simulink model "main_sim"  (R2025b)
settings: Solver=FixedStepAuto  StartTime=0.0  StopTime=100  FixedStep=sample_time  RelTol=1e-3
values from neighbouring files (symbols this model uses):
  A_cut_in = 0.03    [matlab.mat]    (also in params.m = 0.16)
  att_ctrl_time = 0.004    [matlab.mat]    (also in params.m)
  control_allocator_matrix = [0 0 0.106752068321 1.89324793168 0 1 0 0 1 0 0 0 ... (16 elements, 4x4)]    [matlab.mat]    (also in params.m = inv(control_effectiveness_matrix))
  f_xy_tf = load("f_xy_tf.mat").tf1    [params.m]
  initial_euler = [0 0.1 0]    [matlab.mat]    (also in params.m = [0, 0, 0])
  K_coeff = 0.84020150191    [matlab.mat]    (also in params.m = 0.348193185773)
  mav_mass = 0.6    [matlab.mat]    (also in params.m)
  phase_lag = 0    [matlab.mat]    (also in params.m)
  rate_ctrl_time = 0.001    [matlab.mat]    (also in params.m)
  thrust_coeff_bot = 10    [matlab.mat]    (also in params.m = 10.9837)
  thrust_coeff_top = 8.4216    [matlab.mat]    (also in params.m = 9.346)
  top_motor_arm = [0 0 0.1]    [matlab.mat]    (also in params.m = [0, 0, 0.1])
  torque_coeff_bot = 0.1    [matlab.mat]    (also in params.m = 0.1455)
  torque_coeff_top = 1.7735    [matlab.mat]    (also in params.m = 0.2051)
undefined symbols (not defined in the file or in its folder): fractalcoef, SampleTime
libraries: aerolibutil x3, sharedtransform x2, simulink_extras x1, aerolibobsolete x1, matrix_library x1, uavutilslib x1, sensorgpslib x1, mspsensorlib x1
settings Model: Creator=tommy  LastModifiedBy=tommy
settings OptimizationCC: DefaultParameterBehavior=Inlined  UseDivisionForNetSlopeComputation=on  GainParamInheritBuiltInType=on  UseFloatMulNetSlope=on  InlineInvariantSignals=on  EnhancedBackFolding=on  BooleansAsBitfields=on  PassReuseOutputArgsAs=Individual arguments  StateBitsets=on  DataBitsets=on  ZeroExternalMemoryAtStartup=off  ZeroInternalMemoryAtStartup=off  NoFixptDivByZeroProtection=on  EfficientFloat2IntCast=on  LifeSpan=1  OptimizeBlockOrder=speed  DifferentSizesBufferReuse=on  EfficientTunableParamExpr=on
settings DebuggingCC: ParameterTunabilityLossMsg=error
settings HardwareCC: ProdBitPerPointer=32.0  ProdBitPerSizeT=32.0  ProdBitPerPtrDiffT=32.0  ProdLargestAtomicInteger=Long  ProdLargestAtomicFloat=Double  ProdWordSize=32.0  ProdLongLongMode=on  ProdHWDeviceType=ARM Compatible->ARM Cortex-M
settings SFSimCC: MATLABDynamicMemAlloc=off  SimTargetLang=C++  SimDLTargetLibrary=mkl-dnn
settings RTWCC: SystemTargetFile=ert.tlc  TemplateMakefile=ert_default_tmf  TargetLang=C++  Description=Embedded Coder
settings CodeAppCC: ForceParamTrailComments=on  IgnoreCustomStorageClasses=off  OperatorAnnotations=on  SimulinkDataObjDesc=on  SFDataObjDesc=on  CustomSymbolStrGlobalVar=rt$N$M  CustomSymbolStrType=$N$M  CustomSymbolStrFcn=$N$M$F  CustomSymbolStrMacro=$N$M  InsertBlockDesc=on
settings ERTTargetCC: RootIOFormat=Structure reference  ERTCustomFileTemplate=example_file_process.tlc  ERTFilePackagingFormat=CompactWithDataFile  TargetLangStandard=C++11 (ISO)  GenerateSampleERTMain=on  IncludeMdlTerminateFcn=off  CombineSignalStateStructs=on  SuppressErrorStatus=on  SupportAbsoluteTime=off  CodeInterfacePackaging=C++ class  SupportComplex=off

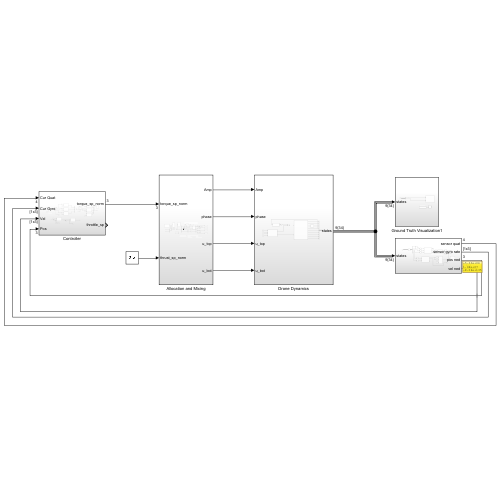
[thumbnail: Simulink's stored preview of the top-level diagram]
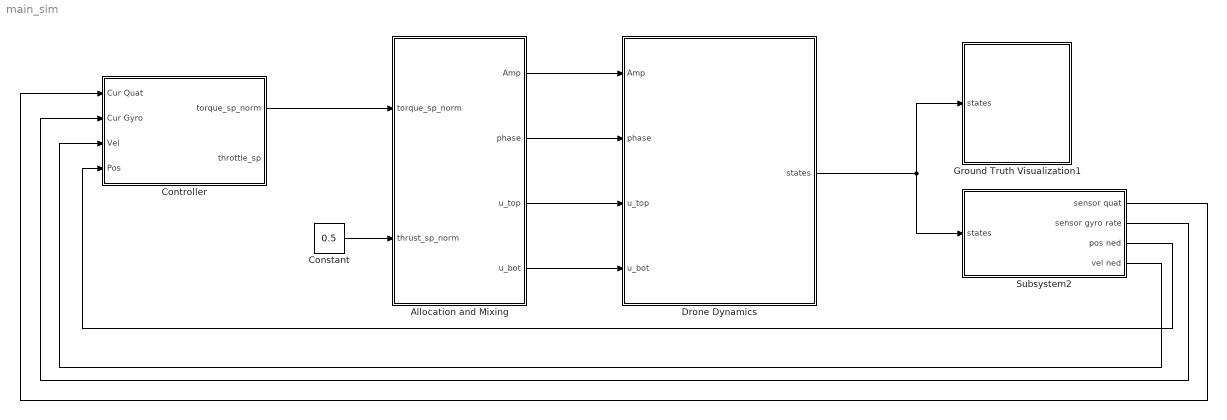
== system main_sim ==
  Allocation and Mixing : Subsystem
  Constant : Constant  Value=0.5
  Controller : Subsystem
  Drone Dynamics : Subsystem
  Ground Truth Visualization1 : Subsystem
  Subsystem2 : Subsystem
  wires:
  Controller/1(torque_sp_norm) -> Allocation and Mixing/1(torque_sp_norm)
  Drone Dynamics/1(states) -> Ground Truth Visualization1/1(states), Subsystem2/1(states)
  Allocation and Mixing/2(phase) -> Drone Dynamics/2(phase)
  Allocation and Mixing/3(u_top) -> Drone Dynamics/3(u_top)
  Allocation and Mixing/4(u_bot) -> Drone Dynamics/4(u_bot)
  Subsystem2/2(sensor gyro rate) -> Controller/2(Cur Gyro)
  Subsystem2/1(sensor quat) -> Controller/1(Cur Quat)
  Allocation and Mixing/1(Amp) -> Drone Dynamics/1(Amp)
  Subsystem2/4(vel ned) -> Controller/3(Vel)
  Subsystem2/3(pos ned) -> Controller/4(Pos)
  Constant/1 -> Allocation and Mixing/2(thrust_sp_norm)

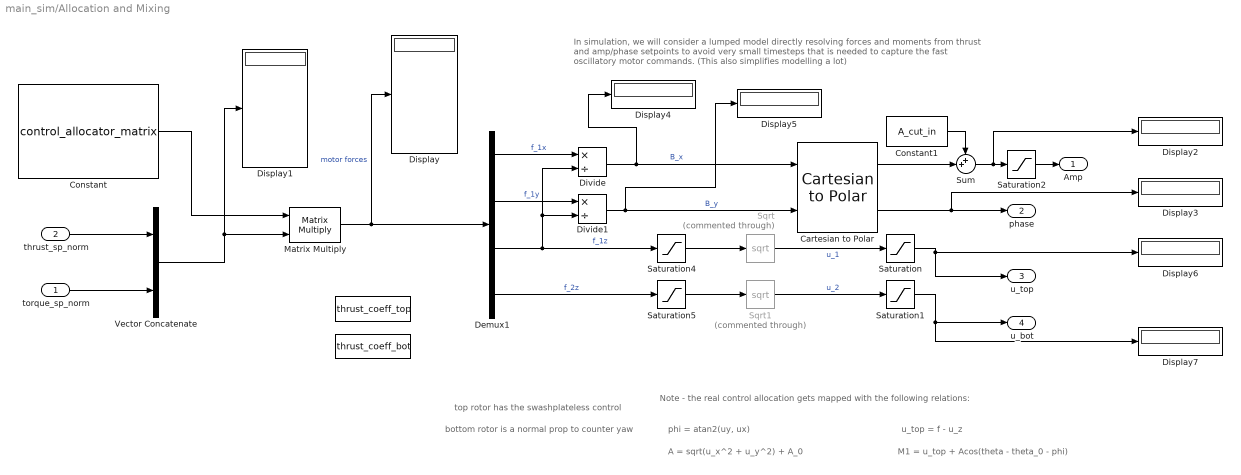
== system main_sim/Allocation and Mixing ==
  note: u_top = f - u_z
  note: In simulation, we will consider a lumped model directly resolving forces and moments from thrust and amp/phase setpoints to avoid very small timesteps that is needed to capture the fast oscillatory motor commands. (This also simplifies modelling a lot)
  note: phi = atan2(uy, ux)
  note: A = sqrt(u_x^2 + u_y^2) + A_0
  note: top rotor has the swashplateless control
  note: bottom rotor is a normal prop to counter yaw
  note: Note - the real control allocation gets mapped with the following relations:
  note: M1 = u_top + Acos(theta - theta_0 - phi)
  torque_sp_norm : Inport
  thrust_sp_norm : Inport  Port=2
  " " : Constant  Value=thrust_coeff_top
  "  " : Constant  Value=thrust_coeff_bot
  Cartesian to Polar : simulink_extras/Transformations/Cartesian to Polar
  Constant : Constant  Value=control_allocator_matrix
  Constant1 : Constant  Value=A_cut_in
  Demux1 : Demux
  Display{,1..7} (8 alike) : Display
  Divide : Product  Inputs=*/
  Divide1 : Product  Inputs=*/
  Matrix Multiply : Product  Multiplication=Matrix(*)
  Saturation : Saturate  UpperLimit=1  LowerLimit=0
  Saturation1 : Saturate  UpperLimit=1  LowerLimit=0
  Saturation2 : Saturate  UpperLimit=0.3
  Saturation4 : Saturate  UpperLimit=inf  LowerLimit=0
  Saturation5 : Saturate  UpperLimit=inf  LowerLimit=0
  Sqrt : Sqrt  Commented=through
  Sqrt1 : Sqrt  Commented=through
  Sum : Sum  Inputs=++|
  Vector Concatenate : Concatenate
  Amp : Outport
  phase : Outport  Port=2
  u_top : Outport  Port=3
  u_bot : Outport  Port=4
  wires:
  Divide/1 -> Display4/1, Cartesian to Polar/1  "B_x"
  Divide1/1 -> Display5/1, Cartesian to Polar/2  "B_y"
  Cartesian to Polar/2 -> Display3/1, phase/1
  Saturation/1 -> u_top/1, Display6/1
  Saturation1/1 -> Display7/1, u_bot/1
  Demux1/1 -> Divide/1  "f_1x"
  Demux1/2 -> Divide1/1  "f_1y"
  Demux1/3 -> Divide/2, Divide1/2, Saturation4/1  "f_1z"
  Demux1/4 -> Saturation5/1  "f_2z"
  Sqrt/1 -> Saturation/1  "u_1"
  Sqrt1/1 -> Saturation1/1  "u_2"
  torque_sp_norm/1 -> Vector Concatenate/2
  Constant/1 -> Matrix Multiply/1
  thrust_sp_norm/1 -> Vector Concatenate/1
  Vector Concatenate/1 -> Display1/1, Matrix Multiply/2
  Matrix Multiply/1 -> Display/1, Demux1/1  "motor forces"
  Sum/1 -> Saturation2/1, Display2/1
  Cartesian to Polar/1 -> Sum/2
  Constant1/1 -> Sum/1
  Saturation4/1 -> Sqrt/1
  Saturation5/1 -> Sqrt1/1
  Saturation2/1 -> Amp/1

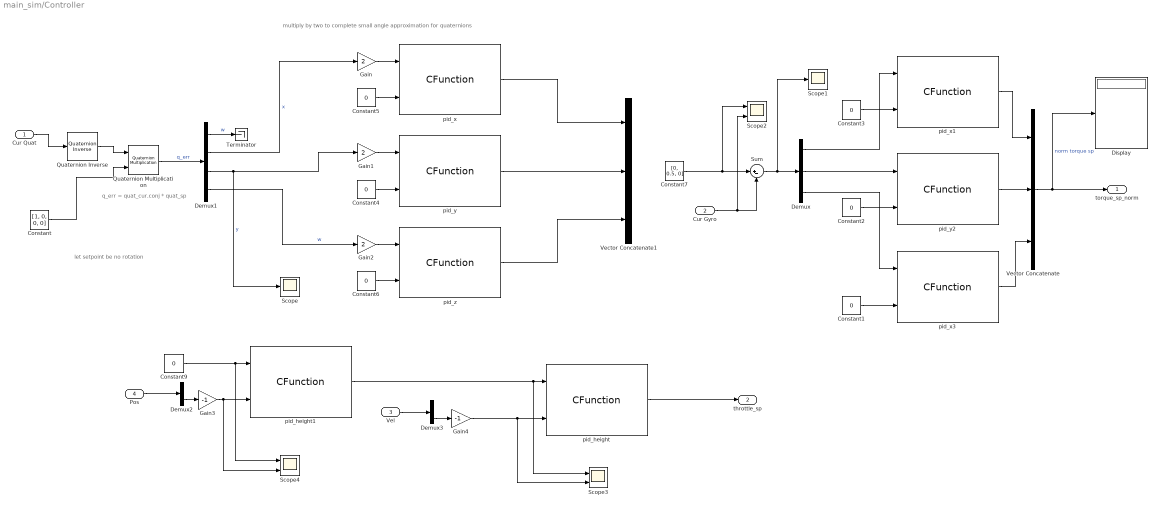
== system main_sim/Controller ==
  note: let setpoint be no rotation
  note: q_err = quat_cur.conj * quat_sp
  note: multiply by two to complete small angle approximation for quaternions
  Cur Quat : Inport
  Cur Gyro : Inport  Port=2
  Vel : Inport  Port=3
  Pos : Inport  Port=4
  Constant : Constant  Value=[1, 0, 0, 0]
  Constant{1..6,9} (7 alike) : Constant  Value=0
  Constant7 : Constant  Value=[0, 0.5, 0]
  Demux : Demux  Outputs=3
  Demux1 : Demux
  Demux2 : Demux  Outputs=3
  Demux3 : Demux  Outputs=3
  Display : Display
  Gain : Gain  Gain=2
  Gain1 : Gain  Gain=2
  Gain2 : Gain  Gain=2
  Gain3 : Gain  Gain=-1
  Gain4 : Gain  Gain=-1
  Quaternion Inverse : aerolibutil/Quaternion Inverse
  Quaternion Multiplication : aerolibutil/Quaternion Multiplication
  Scope : Scope
      settings: ActiveDisplayYMinimum=-0.059979169270678333  ActiveDisplayYMaximum=-0.039979169270678329  DataLoggingVariableName=ScopeData2
  Scope1 : Scope
      settings: ActiveDisplayYMinimum=-0.0842010868455836  ActiveDisplayYMaximum=-0.046176733596834114  DataLoggingVariableName=ScopeData3
  Scope2 : Scope  NumInputPorts=2
      settings: ActiveDisplayYMinimum=-2.2288514415526066  ActiveDisplayYMaximum=0.61387387896787893  DataLoggingVariableName=ScopeData4
  Scope3 : Scope  NumInputPorts=2
      settings: ActiveDisplayYMinimum=-1.8084870099704817  ActiveDisplayYMaximum=0.34454279174231495  DataLoggingVariableName=ScopeData6
  Scope4 : Scope  NumInputPorts=2
      settings: ActiveDisplayYMinimum=-2.2966254517668858  ActiveDisplayYMaximum=2.4973444218048826  DataLoggingVariableName=ScopeData7
  Sum : Sum  Inputs=|+-
  Terminator : Terminator
  Vector Concatenate : Concatenate  NumInputs=3
  Vector Concatenate1 : Concatenate  NumInputs=3
  pid_height : CFunction  OutputCode=|  StartCode=obj_ptr = create_pid((float)Ts, (float)max, (float)min, (float)K, (float)Kp, (float)Ki, (float)Kd, (float)clamp, (float)alpha);  TerminateCode=|  CodegenOutputCode=|  CodegenStartCode=obj_ptr = create_pid((float)Ts, (float)max, (float)min, (float)K, (float)Kp, (float)Ki, (float)Kd, (float)clamp, (float)alpha);  CodegenTerminateCode=|  SampleTime=SampleTime  SimCustomHeaderFile="#include \"cpp/pid_wrap.hpp\""  SimCustomSourceFile=pid_wrap.cpp  CustomHeaderFile="#include \"cpp/pid_wrap.hpp\""  CustomSourceFile=pid_wrap.cpp  CustomCodeIsMultiInstantiable=on  Ts=att_ctrl_time  max=1  min=0.1  K=1  Kp=0.3  Ki=0.6  Kd=0  clamp=0.8  alpha=0  SampleTime=att_ctrl_time
      OutputCode=|
      | if (obj_ptr != 0) {
      |     out = (double)run_pid(obj_ptr, (float)setpoint, (float)measurement);
      | }
      TerminateCode=|
      | if (obj_ptr != 0) {
      |     delete_pid(obj_ptr);
      |     obj_ptr = 0;
      | }
      CodegenOutputCode=|
      | if (obj_ptr != 0) {
      |     out = (double)run_pid(obj_ptr, (float)setpoint, (float)measurement);
      | }
      CodegenTerminateCode=|
      | if (obj_ptr != 0) {
      |     delete_pid(obj_ptr);
      |     obj_ptr = 0;
      | }
  pid_height1 : CFunction  OutputCode=|  StartCode=obj_ptr = create_pid((float)Ts, (float)max, (float)min, (float)K, (float)Kp, (float)Ki, (float)Kd, (float)clamp, (float)alpha);  TerminateCode=|  CodegenOutputCode=|  CodegenStartCode=obj_ptr = create_pid((float)Ts, (float)max, (float)min, (float)K, (float)Kp, (float)Ki, (float)Kd, (float)clamp, (float)alpha);  CodegenTerminateCode=|  SampleTime=SampleTime  SimCustomHeaderFile="#include \"cpp/pid_wrap.hpp\""  SimCustomSourceFile=pid_wrap.cpp  CustomHeaderFile="#include \"cpp/pid_wrap.hpp\""  CustomSourceFile=pid_wrap.cpp  CustomCodeIsMultiInstantiable=on  Ts=att_ctrl_time  max=5  min=-5  K=1  Kp=0.2  Ki=0  Kd=0  clamp=0.8  alpha=0  SampleTime=att_ctrl_time
      OutputCode=|
      | if (obj_ptr != 0) {
      |     out = (double)run_pid(obj_ptr, (float)setpoint, (float)measurement);
      | }
      TerminateCode=|
      | if (obj_ptr != 0) {
      |     delete_pid(obj_ptr);
      |     obj_ptr = 0;
      | }
      CodegenOutputCode=|
      | if (obj_ptr != 0) {
      |     out = (double)run_pid(obj_ptr, (float)setpoint, (float)measurement);
      | }
      CodegenTerminateCode=|
      | if (obj_ptr != 0) {
      |     delete_pid(obj_ptr);
      |     obj_ptr = 0;
      | }
  pid_x : CFunction  OutputCode=|  StartCode=obj_ptr = create_pid((float)Ts, (float)max, (float)min, (float)K, (float)Kp, (float)Ki, (float)Kd, (float)clamp, (float)alpha);  TerminateCode=|  CodegenOutputCode=|  CodegenStartCode=obj_ptr = create_pid((float)Ts, (float)max, (float)min, (float)K, (float)Kp, (float)Ki, (float)Kd, (float)clamp, (float)alpha);  CodegenTerminateCode=|  SampleTime=SampleTime  SimCustomHeaderFile="#include \"cpp/pid_wrap.hpp\""  SimCustomSourceFile=pid_wrap.cpp  CustomHeaderFile="#include \"cpp/pid_wrap.hpp\""  CustomSourceFile=pid_wrap.cpp  CustomCodeIsMultiInstantiable=on  Ts=att_ctrl_time  max=1  min=-1  K=1  Kp=0.1  Ki=0  Kd=0  clamp=0  alpha=0  SampleTime=att_ctrl_time
      OutputCode=|
      | if (obj_ptr != 0) {
      |     out = (double)run_pid(obj_ptr, (float)setpoint, (float)measurement);
      | }
      TerminateCode=|
      | if (obj_ptr != 0) {
      |     delete_pid(obj_ptr);
      |     obj_ptr = 0;
      | }
      CodegenOutputCode=|
      | if (obj_ptr != 0) {
      |     out = (double)run_pid(obj_ptr, (float)setpoint, (float)measurement);
      | }
      CodegenTerminateCode=|
      | if (obj_ptr != 0) {
      |     delete_pid(obj_ptr);
      |     obj_ptr = 0;
      | }
  pid_x1 : CFunction  OutputCode=|  StartCode=obj_ptr = create_pid((float)Ts, (float)max, (float)min, (float)K, (float)Kp, (float)Ki, (float)Kd, (float)clamp, (float)alpha);  TerminateCode=|  CodegenOutputCode=|  CodegenStartCode=obj_ptr = create_pid((float)Ts, (float)max, (float)min, (float)K, (float)Kp, (float)Ki, (float)Kd, (float)clamp, (float)alpha);  CodegenTerminateCode=|  SampleTime=SampleTime  SimCustomHeaderFile="#include \"cpp/pid_wrap.hpp\""  SimCustomSourceFile=pid_wrap.cpp  CustomHeaderFile="#include \"cpp/pid_wrap.hpp\""  CustomSourceFile=pid_wrap.cpp  CustomCodeIsMultiInstantiable=on  Ts=rate_ctrl_time  max=1  min=-1  K=1  Kp=0.02  Ki=0  Kd=0  clamp=0  alpha=0  SampleTime=rate_ctrl_time
      OutputCode=|
      | if (obj_ptr != 0) {
      |     out = (double)run_pid(obj_ptr, (float)setpoint, (float)measurement);
      | }
      TerminateCode=|
      | if (obj_ptr != 0) {
      |     delete_pid(obj_ptr);
      |     obj_ptr = 0;
      | }
      CodegenOutputCode=|
      | if (obj_ptr != 0) {
      |     out = (double)run_pid(obj_ptr, (float)setpoint, (float)measurement);
      | }
      CodegenTerminateCode=|
      | if (obj_ptr != 0) {
      |     delete_pid(obj_ptr);
      |     obj_ptr = 0;
      | }
  pid_x3 : CFunction  OutputCode=|  StartCode=obj_ptr = create_pid((float)Ts, (float)max, (float)min, (float)K, (float)Kp, (float)Ki, (float)Kd, (float)clamp, (float)alpha);  TerminateCode=|  CodegenOutputCode=|  CodegenStartCode=obj_ptr = create_pid((float)Ts, (float)max, (float)min, (float)K, (float)Kp, (float)Ki, (float)Kd, (float)clamp, (float)alpha);  CodegenTerminateCode=|  SampleTime=SampleTime  SimCustomHeaderFile="#include \"cpp/pid_wrap.hpp\""  SimCustomSourceFile=pid_wrap.cpp  CustomHeaderFile="#include \"cpp/pid_wrap.hpp\""  CustomSourceFile=pid_wrap.cpp  CustomCodeIsMultiInstantiable=on  Ts=rate_ctrl_time  max=1  min=-1  K=1  Kp=0.1  Ki=0.3  Kd=0  clamp=0.3  alpha=0  SampleTime=rate_ctrl_time
      OutputCode=|
      | if (obj_ptr != 0) {
      |     out = (double)run_pid(obj_ptr, (float)setpoint, (float)measurement);
      | }
      TerminateCode=|
      | if (obj_ptr != 0) {
      |     delete_pid(obj_ptr);
      |     obj_ptr = 0;
      | }
      CodegenOutputCode=|
      | if (obj_ptr != 0) {
      |     out = (double)run_pid(obj_ptr, (float)setpoint, (float)measurement);
      | }
      CodegenTerminateCode=|
      | if (obj_ptr != 0) {
      |     delete_pid(obj_ptr);
      |     obj_ptr = 0;
      | }
  pid_y : CFunction  OutputCode=|  StartCode=obj_ptr = create_pid((float)Ts, (float)max, (float)min, (float)K, (float)Kp, (float)Ki, (float)Kd, (float)clamp, (float)alpha);  TerminateCode=|  CodegenOutputCode=|  CodegenStartCode=obj_ptr = create_pid((float)Ts, (float)max, (float)min, (float)K, (float)Kp, (float)Ki, (float)Kd, (float)clamp, (float)alpha);  CodegenTerminateCode=|  SampleTime=SampleTime  SimCustomHeaderFile="#include \"cpp/pid_wrap.hpp\""  SimCustomSourceFile=pid_wrap.cpp  CustomHeaderFile="#include \"cpp/pid_wrap.hpp\""  CustomSourceFile=pid_wrap.cpp  CustomCodeIsMultiInstantiable=on  Ts=att_ctrl_time  max=1  min=-1  K=1  Kp=0.5  Ki=0  Kd=0  clamp=0  alpha=0  SampleTime=att_ctrl_time
      OutputCode=|
      | if (obj_ptr != 0) {
      |     out = (double)run_pid(obj_ptr, (float)setpoint, (float)measurement);
      | }
      TerminateCode=|
      | if (obj_ptr != 0) {
      |     delete_pid(obj_ptr);
      |     obj_ptr = 0;
      | }
      CodegenOutputCode=|
      | if (obj_ptr != 0) {
      |     out = (double)run_pid(obj_ptr, (float)setpoint, (float)measurement);
      | }
      CodegenTerminateCode=|
      | if (obj_ptr != 0) {
      |     delete_pid(obj_ptr);
      |     obj_ptr = 0;
      | }
  pid_y2 : CFunction  OutputCode=|  StartCode=obj_ptr = create_pid((float)Ts, (float)max, (float)min, (float)K, (float)Kp, (float)Ki, (float)Kd, (float)clamp, (float)alpha);  TerminateCode=|  CodegenOutputCode=|  CodegenStartCode=obj_ptr = create_pid((float)Ts, (float)max, (float)min, (float)K, (float)Kp, (float)Ki, (float)Kd, (float)clamp, (float)alpha);  CodegenTerminateCode=|  SampleTime=SampleTime  SimCustomHeaderFile="#include \"cpp/pid_wrap.hpp\""  SimCustomSourceFile=pid_wrap.cpp  CustomHeaderFile="#include \"cpp/pid_wrap.hpp\""  CustomSourceFile=pid_wrap.cpp  CustomCodeIsMultiInstantiable=on  Ts=rate_ctrl_time  max=1  min=-1  K=1  Kp=0.02  Ki=0  Kd=0  clamp=0  alpha=0  SampleTime=rate_ctrl_time
      OutputCode=|
      | if (obj_ptr != 0) {
      |     out = (double)run_pid(obj_ptr, (float)setpoint, (float)measurement);
      | }
      TerminateCode=|
      | if (obj_ptr != 0) {
      |     delete_pid(obj_ptr);
      |     obj_ptr = 0;
      | }
      CodegenOutputCode=|
      | if (obj_ptr != 0) {
      |     out = (double)run_pid(obj_ptr, (float)setpoint, (float)measurement);
      | }
      CodegenTerminateCode=|
      | if (obj_ptr != 0) {
      |     delete_pid(obj_ptr);
      |     obj_ptr = 0;
      | }
  pid_z : CFunction  OutputCode=|  StartCode=obj_ptr = create_pid((float)Ts, (float)max, (float)min, (float)K, (float)Kp, (float)Ki, (float)Kd, (float)clamp, (float)alpha);  TerminateCode=|  CodegenOutputCode=|  CodegenStartCode=obj_ptr = create_pid((float)Ts, (float)max, (float)min, (float)K, (float)Kp, (float)Ki, (float)Kd, (float)clamp, (float)alpha);  CodegenTerminateCode=|  SampleTime=SampleTime  SimCustomHeaderFile="#include \"cpp/pid_wrap.hpp\""  SimCustomSourceFile=pid_wrap.cpp  CustomHeaderFile="#include \"cpp/pid_wrap.hpp\""  CustomSourceFile=pid_wrap.cpp  CustomCodeIsMultiInstantiable=on  Ts=att_ctrl_time  max=1  min=-1  K=1  Kp=0.1  Ki=0  Kd=0  clamp=0  alpha=0  SampleTime=att_ctrl_time
      OutputCode=|
      | if (obj_ptr != 0) {
      |     out = (double)run_pid(obj_ptr, (float)setpoint, (float)measurement);
      | }
      TerminateCode=|
      | if (obj_ptr != 0) {
      |     delete_pid(obj_ptr);
      |     obj_ptr = 0;
      | }
      CodegenOutputCode=|
      | if (obj_ptr != 0) {
      |     out = (double)run_pid(obj_ptr, (float)setpoint, (float)measurement);
      | }
      CodegenTerminateCode=|
      | if (obj_ptr != 0) {
      |     delete_pid(obj_ptr);
      |     obj_ptr = 0;
      | }
  torque_sp_norm : Outport
  throttle_sp : Outport  Port=2
  wires:
  Cur Gyro/1 -> Scope2/2, Sum/2
  Sum/1 -> Scope1/1, Demux/1
  Demux/1 -> pid_x1/1
  Demux/2 -> pid_y2/1
  Demux/3 -> pid_x3/1
  Constant1/1 -> pid_x3/2
  Constant2/1 -> pid_y2/2
  Constant3/1 -> pid_x1/2
  pid_x1/1 -> Vector Concatenate/1
  pid_y2/1 -> Vector Concatenate/2
  Vector Concatenate/1 -> Display/1, torque_sp_norm/1  "norm torque sp"
  Constant6/1 -> pid_z/2
  Constant/1 -> Quaternion Multiplication/2
  Gain2/1 -> pid_z/1
  pid_y/1 -> Vector Concatenate1/2
  Quaternion Inverse/1 -> Quaternion Multiplication/1
  Cur Quat/1 -> Quaternion Inverse/1
  Gain1/1 -> pid_y/1
  Constant5/1 -> pid_x/2
  pid_x/1 -> Vector Concatenate1/1
  pid_z/1 -> Vector Concatenate1/3
  Gain/1 -> pid_x/1
  Quaternion Multiplication/1 -> Demux1/1  "q_err"
  Constant4/1 -> pid_y/2
  Demux1/1 -> Terminator/1  "w"
  Demux1/2 -> Gain/1  "x"
  Demux1/3 -> Scope/1, Gain1/1  "y"
  Demux1/4 -> Gain2/1  "w"
  Constant7/1 -> Scope2/1, Sum/1
  pid_height/1 -> throttle_sp/1
  Vel/1 -> Demux3/1
  Demux3/3 -> Gain4/1
  Gain4/1 -> Scope3/2, pid_height/2
  Demux2/3 -> Gain3/1
  Pos/1 -> Demux2/1
  Gain3/1 -> pid_height1/2, Scope4/2
  Constant9/1 -> pid_height1/1, Scope4/1
  pid_height1/1 -> Scope3/1, pid_height/1
  pid_x3/1 -> Vector Concatenate/3

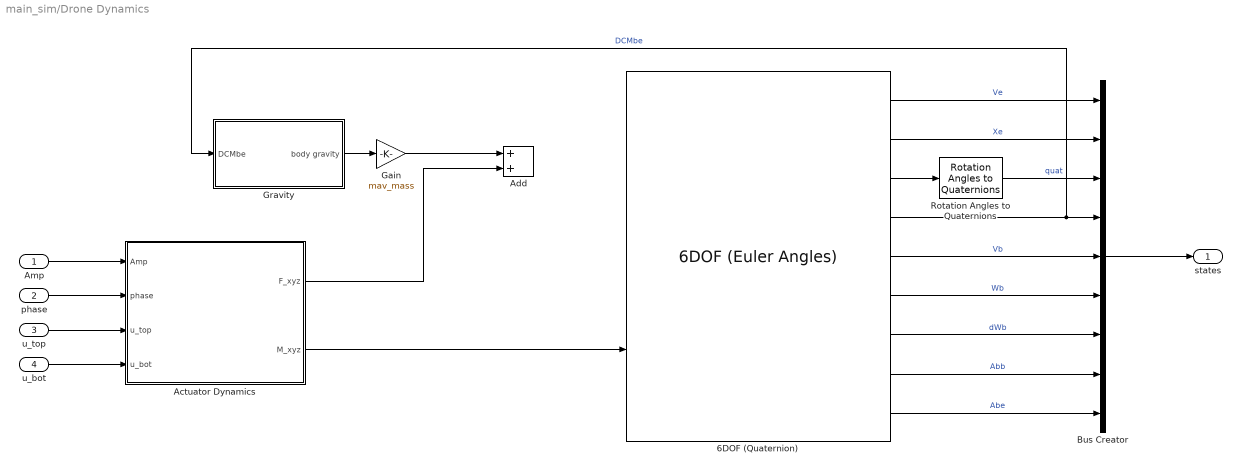
== system main_sim/Drone Dynamics ==
  Amp : Inport
  phase : Inport  Port=2
  u_top : Inport  Port=3
  u_bot : Inport  Port=4
  6DOF (Quaternion) : aerolibobsolete/6DOF (Euler Angles)  units=Metric (MKS)  mtype=Fixed  rep=Quaternion  xme_0=[0 0 0]  Vm_0=[0 0 0]  eul_0=initial_euler  pm_0=[0 0.2 0]  mass_0=mav_mass  mass_e=0.5  mass_f=2.0  inertia=mav_inertia  inertia_e=eye(3)  inertia_f=2*eye(3)  k_quat=1.0  vre_flag=on  abi_flag=on  aMode=0  xme_statename=''  Vm_statename=''  eul_statename=''  quat_statename=''  pm_statename=''  mass_statename=''
  Actuator Dynamics : Subsystem
  Add : Sum
  Bus Creator : BusCreator  Inputs=9
  Gain : Gain  Gain=mav_mass
  Gravity : Subsystem
  Rotation Angles to Quaternions : sharedtransform/Rotation Angles to Quaternions  rotationOrder=XYZ  aMode=aMode
  states : Outport
  wires:
  6DOF (Quaternion)/7 -> Bus Creator/7  "dWb"
  u_top/1 -> Actuator Dynamics/3(u_top)
  6DOF (Quaternion)/8 -> Bus Creator/8  "Abb"
  6DOF (Quaternion)/6 -> Bus Creator/6  "Wb"
  Rotation Angles to Quaternions/1 -> Bus Creator/3  "quat"
  u_bot/1 -> Actuator Dynamics/4(u_bot)
  Bus Creator/1 -> states/1
  6DOF (Quaternion)/9 -> Bus Creator/9  "Abe"
  phase/1 -> Actuator Dynamics/2(phase)
  Actuator Dynamics/2(M_xyz) -> 6DOF (Quaternion)/2
  6DOF (Quaternion)/1 -> Bus Creator/1  "Ve"
  6DOF (Quaternion)/2 -> Bus Creator/2  "Xe"
  Amp/1 -> Actuator Dynamics/1(Amp)
  6DOF (Quaternion)/5 -> Bus Creator/5  "Vb"
  6DOF (Quaternion)/4 -> Bus Creator/4, Gravity/1(DCMbe)  "DCMbe"
  6DOF (Quaternion)/3 -> Rotation Angles to Quaternions/1
  Actuator Dynamics/1(F_xyz) -> Add/2
  Gravity/1(body gravity) -> Gain/1
  Gain/1 -> Add/1

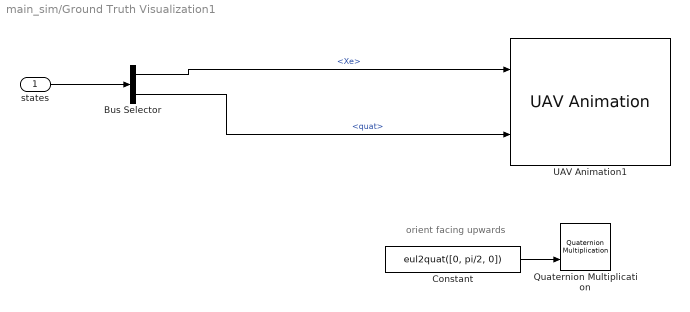
== system main_sim/Ground Truth Visualization1 ==
  note: orient facing upwards
  states : Inport
  Bus Selector : BusSelector  OutputSignals=Xe,quat
  Constant : Constant  Value=eul2quat([0, pi/2, 0])  VectorParams1D=off
  Quaternion Multiplication : aerolibutil/Quaternion Multiplication
  UAV Animation1 : uavutilslib/UAV Animation  NumUAV=1  DynamicUAVConfig=off  UAVType=Multirotor  UAVSize=1  UAVColor=[1 0 0]  UAVTrajectoryAlpha=1  InertialZDirection=Down  RotationFormat=Quaternion  DrawMarkers=off  SampleTime=0.05
  wires:
  states/1 -> Bus Selector/1
  Bus Selector/1 -> UAV Animation1/1  "<Xe>"
  Bus Selector/2 -> UAV Animation1/2  "<quat>"
  Constant/1 -> Quaternion Multiplication/2

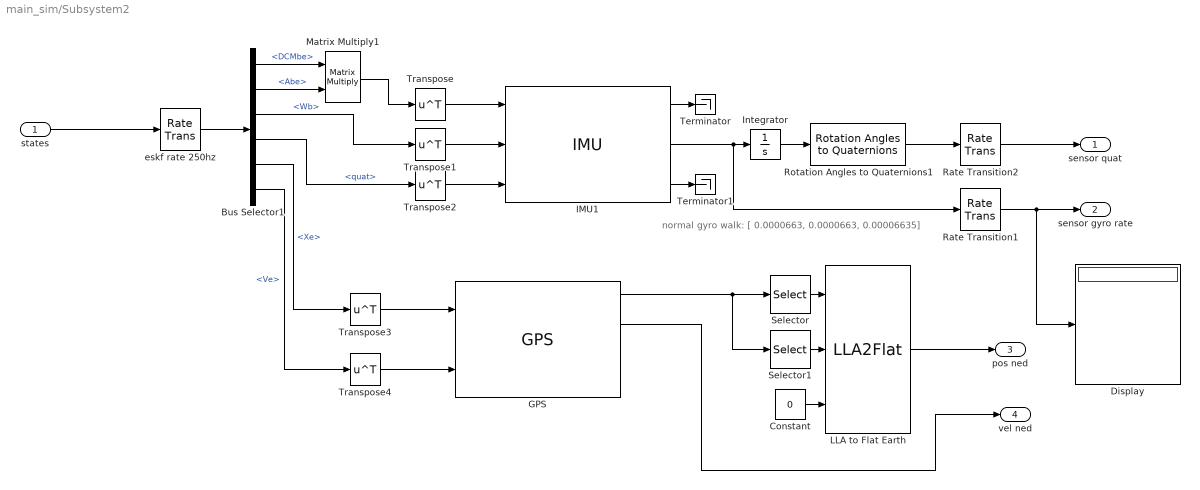
== system main_sim/Subsystem2 ==
  note: normal gyro walk: [ 0.0000663, 0.0000663, 0.00006635]
  states : Inport
  Bus Selector1 : BusSelector  OutputSignals=DCMbe,Abe,Wb,quat,Xe,Ve
  Constant : Constant  Value=0
  Display : Display
  GPS : sensorgpslib/GPS  DispRefFrame=NED  PositionInputFormat=Local  ReferenceLocation=[ 43.660624994362166, -79.39579849130422, 0 ]  HorizontalPositionAccuracy=1.6  VerticalPositionAccuracy=2  VelocityAccuracy=0.1  DecayFactor=0.999  SeedDouble=67  SimulateUsing=Interpreted execution
      settings: LibrarySourceBlock=uavsimlib/GPS
  IMU1 : mspsensorlib/IMU  DispRefFrame=NED  TemperaturePort=off  Temperature=0  MagneticFieldPort=off  MagneticFieldNED=[ 27.5550, -2.4169, -16.0849 ]  MagneticFieldENU=[ -2.4169, 27.5550, 16.0849 ]  SeedDouble=67  SimulateUsing=Interpreted execution  AccelParamsMeasurementRange=Inf  AccelParamsResolution=0  AccelParamsConstantBias=[ 0, 0, 0 ]  AccelParamsAxesMisalignment=[ 1, 0, 0; 0, 1, 0; 0, 0, 1 ]  AccelParamsNoiseDensity=[ 0, 0, 0 ]  AccelParamsBiasInstability=[ 0, 0, 0 ]  AccelParamsBiasInstabilityNumerator=fractalcoef().Numerator  AccelParamsBiasInstabilityDenominator=fractalcoef().Denominator  AccelParamsRandomWalk=[ 0, 0, 0 ]  AccelParamsNoiseType=double-sided  AccelParamsTemperatureBias=[ 0, 0, 0 ]  AccelParamsTemperatureScaleFactor=[ 0, 0, 0 ]  GyroParamsMeasurementRange=Inf  GyroParamsResolution=0  GyroParamsConstantBias=[ 0, 0, 0 ]  GyroParamsAxesMisalignment=[ 100, 0, 0; 0, 100, 0; 0, 0, 100 ]  GyroParamsAccelerationBias=[ 0, 0, 0 ]  GyroParamsNoiseDensity=[0, 0, 0]  GyroParamsBiasInstability=[ 0, 0, 0 ]  GyroParamsBiasInstabilityNumerator=fractalcoef().Numerator  GyroParamsBiasInstabilityDenominator=fractalcoef().Denominator  GyroParamsRandomWalk=[ 0, 0, 0 ]  GyroParamsNoiseType=double-sided  GyroParamsTemperatureBias=[ 0, 0, 0 ]  GyroParamsTemperatureScaleFactor=[ 0, 0, 0 ]  MagParamsMeasurementRange=Inf  MagParamsResolution=0  MagParamsConstantBias=[ 0, 0, 0 ]  MagParamsAxesMisalignment=[ 100, 0, 0; 0, 100, 0; 0, 0, 100 ]  MagParamsNoiseDensity=[ 0, 0, 0 ]  MagParamsBiasInstability=[ 0, 0, 0 ]  MagParamsBiasInstabilityNumerator=fractalcoef().Numerator  MagParamsBiasInstabilityDenominator=fractalcoef().Denominator  MagParamsRandomWalk=[ 0, 0, 0 ]  MagParamsNoiseType=double-sided  MagParamsTemperatureBias=[ 0, 0, 0 ]  MagParamsTemperatureScaleFactor=[ 0, 0, 0 ]
  Integrator : Integrator  InitialCondition=initial_euler
  LLA to Flat Earth : LLA2Flat  LL0=[43.660624994362166, -79.39579849130422]
  Matrix Multiply1 : Product  Multiplication=Matrix(*)
  Rate Transition1 : RateTransition  OutPortSampleTime=1/1000
  Rate Transition2 : RateTransition  OutPortSampleTime=1/250
  Rotation Angles to Quaternions1 : sharedtransform/Rotation Angles to Quaternions  rotationOrder=XYZ  aMode=aMode
  Selector : Selector  InputPortWidth=3  IndexOptions=Index vector (dialog)  Indices=[1 2]  OutputSizes=1
  Selector1 : Selector  InputPortWidth=3  IndexOptions=Index vector (dialog)  Indices=[3]  OutputSizes=1
  Terminator : Terminator
  Terminator1 : Terminator
  Transpose{,1..4} (5 alike) : Math  Operator=transpose
  eskf rate 250hz : RateTransition  OutPortSampleTime=1/250
  sensor quat : Outport
  sensor gyro rate : Outport  Port=2
  pos ned : Outport  Port=3
  vel ned : Outport  Port=4
  wires:
  Transpose1/1 -> IMU1/2
  IMU1/2 -> Integrator/1, Rate Transition1/1
  Matrix Multiply1/1 -> Transpose/1
  Transpose/1 -> IMU1/1
  Integrator/1 -> Rotation Angles to Quaternions1/1
  Transpose2/1 -> IMU1/3
  Bus Selector1/4 -> Transpose2/1  "<quat>"
  Bus Selector1/3 -> Transpose1/1  "<Wb>"
  Rotation Angles to Quaternions1/1 -> Rate Transition2/1
  states/1 -> eskf rate 250hz/1
  eskf rate 250hz/1 -> Bus Selector1/1
  IMU1/1 -> Terminator/1
  IMU1/3 -> Terminator1/1
  Bus Selector1/1 -> Matrix Multiply1/1  "<DCMbe>"
  Bus Selector1/2 -> Matrix Multiply1/2  "<Abe>"
  Rate Transition1/1 -> Display/1, sensor gyro rate/1
  Rate Transition2/1 -> sensor quat/1
  GPS/1 -> Selector1/1, Selector/1
  Selector/1 -> LLA to Flat Earth/1
  Selector1/1 -> LLA to Flat Earth/2
  Constant/1 -> LLA to Flat Earth/3
  GPS/2 -> vel ned/1
  LLA to Flat Earth/1 -> pos ned/1
  Bus Selector1/6 -> Transpose4/1  "<Ve>"
  Bus Selector1/5 -> Transpose3/1  "<Xe>"
  Transpose3/1 -> GPS/1
  Transpose4/1 -> GPS/2

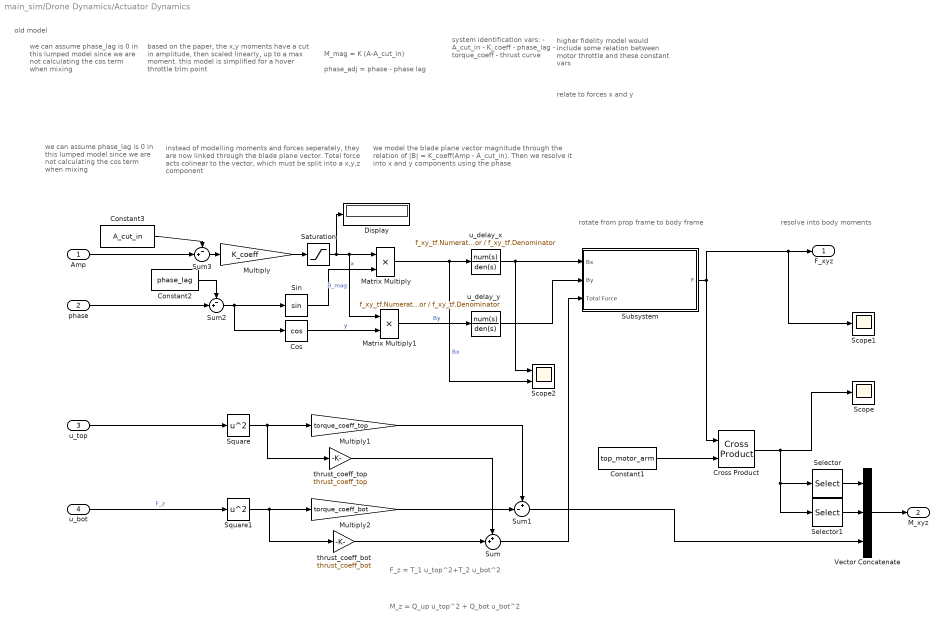
== system main_sim/Drone Dynamics/Actuator Dynamics ==
  note: old model
  note: relate to forces x and y
  note: we can assume phase_lag is 0 in this lumped model since we are not calculating the cos term when mixing
  note: higher fidelity model would include some relation between motor throttle and these constant vars
  note: system identification vars:
      | - A_cut_in
      | - K_coeff
      | - phase_lag
      | - torque_coeff
      | - thrust curve
  note: M_mag = K (A-A_cut_in)
  note: based on the paper, the x,y moments have a cut in amplitude, then scaled linearly, up to a max moment. this model is simplified for a hover throttle trim point
  note: phase_adj = phase - phase lag
  note: M_z = Q_up u_top^2 + Q_bot u_bot^2
  note: F_z = T_1 u_top^2+T_2 u_bot^2
  note: resolve into body moments
  note: we can assume phase_lag is 0 in this lumped model since we are not calculating the cos term when mixing
  note: instead of modelling moments and forces seperately, they are now linked through the blade plane vector. Total force acts colinear to the vector, which must be split into a x,y,z component
  note: we model the blade plane vector magnitude through the relation of |B| = K_coeff(Amp - A_cut_in). Then we resolve it into x and y components using the phase
  note: rotate from prop frame to body frame
  Amp : Inport
  phase : Inport  Port=2
  u_top : Inport  Port=3
  u_bot : Inport  Port=4
  Constant1 : Constant  Value=top_motor_arm
  Constant2 : Constant  Value=phase_lag
  Constant3 : Constant  Value=A_cut_in
  Cos : Trigonometry  Operator=cos
  Cross Product : matrix_library/Cross Product
  Display : Display
  Matrix Multiply : Product
  Matrix Multiply1 : Product
  Multiply : Gain  Gain=K_coeff
  Multiply1 : Gain  Gain=torque_coeff_top
  Multiply2 : Gain  Gain=torque_coeff_bot
  Saturation : Saturate  UpperLimit=inf  LowerLimit=0
  Scope : Scope
      settings: ActiveDisplayYMinimum=-0.0046517365862840283  ActiveDisplayYMaximum=0.012758813227963812
  Scope1 : Scope
      settings: ActiveDisplayYMinimum=-1  ActiveDisplayYMaximum=1
  Scope2 : Scope  NumInputPorts=2
      settings: ActiveDisplayYMinimum=-0.92569474928807993  ActiveDisplayYMaximum=0.036339446893860372  DataLoggingVariableName=ScopeData5
  Selector : Selector  InputPortWidth=3  IndexOptions=Index vector (dialog)  Indices=[1]  OutputSizes=1
  Selector1 : Selector  InputPortWidth=3  IndexOptions=Index vector (dialog)  Indices=[2]  OutputSizes=1
  Sin : Trigonometry
  Square : Math  Operator=square
  Square1 : Math  Operator=square
  Subsystem : Subsystem
  Sum : Sum  Inputs=++|
  Sum1 : Sum  Inputs=+-|
  Sum2 : Sum  Inputs=-+|
  Sum3 : Sum  Inputs=-+|
  Vector Concatenate : Concatenate  NumInputs=3
  thrust_coeff_bot : Gain  Gain=thrust_coeff_bot
  thrust_coeff_top : Gain  Gain=thrust_coeff_top
  u_delay_x : TransferFcn  Numerator=f_xy_tf.Numerator  Denominator=f_xy_tf.Denominator
  u_delay_y : TransferFcn  Numerator=f_xy_tf.Numerator  Denominator=f_xy_tf.Denominator
  F_xyz : Outport
  M_xyz : Outport  Port=2
  wires:
  u_bot/1 -> Square1/1  "F_z"
  Constant2/1 -> Sum2/1
  phase/1 -> Sum2/2
  Sum2/1 -> Cos/1, Sin/1
  Amp/1 -> Sum3/2
  Constant3/1 -> Sum3/1
  Sum3/1 -> Multiply/1
  Multiply/1 -> Saturation/1
  Matrix Multiply/1 -> Scope2/2, u_delay_x/1  "Bx"
  Sin/1 -> Matrix Multiply/2  "x"
  Matrix Multiply1/1 -> u_delay_y/1  "By"
  Cos/1 -> Matrix Multiply1/2  "y"
  Saturation/1 -> Display/1, Matrix Multiply1/1, Matrix Multiply/1  "B_mag"
  u_top/1 -> Square/1
  Constant1/1 -> Cross Product/2
  Cross Product/1 -> Selector1/1, Selector/1, Scope/1
  Sum/1 -> Subsystem/3(Total Force)
  Subsystem/1(F) -> Scope1/1, F_xyz/1, Cross Product/1
  Square/1 -> thrust_coeff_top/1, Multiply1/1
  u_delay_y/1 -> Subsystem/2(By)
  u_delay_x/1 -> Scope2/1, Subsystem/1(Bx)
  thrust_coeff_top/1 -> Sum/1
  thrust_coeff_bot/1 -> Sum/2
  Vector Concatenate/1 -> M_xyz/1
  Selector/1 -> Vector Concatenate/1
  Selector1/1 -> Vector Concatenate/2
  Multiply1/1 -> Sum1/1
  Multiply2/1 -> Sum1/2
  Square1/1 -> Multiply2/1, thrust_coeff_bot/1
  Sum1/1 -> Vector Concatenate/3

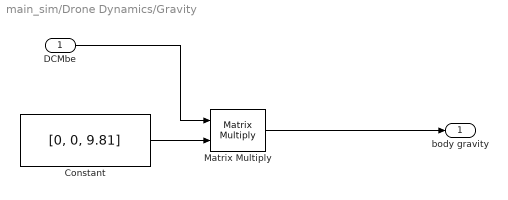
== system main_sim/Drone Dynamics/Gravity ==
  DCMbe : Inport
  Constant : Constant  Value=[0, 0, 9.81]
  Matrix Multiply : Product  Multiplication=Matrix(*)
  body gravity : Outport
  wires:
  DCMbe/1 -> Matrix Multiply/1
  Constant/1 -> Matrix Multiply/2
  Matrix Multiply/1 -> body gravity/1

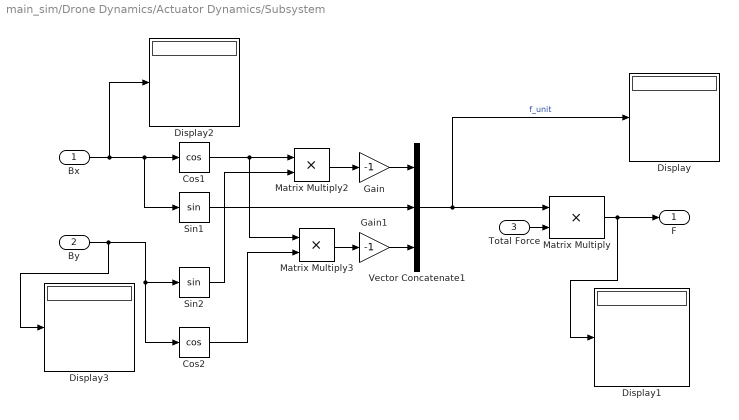
== system main_sim/Drone Dynamics/Actuator Dynamics/Subsystem ==
  Bx : Inport
  By : Inport  Port=2
  Total Force : Inport  Port=3
  Cos1 : Trigonometry  Operator=cos
  Cos2 : Trigonometry  Operator=cos
  Display{,1..3} (4 alike) : Display
  Gain : Gain  Gain=-1
  Gain1 : Gain  Gain=-1
  Matrix Multiply : Product
  Matrix Multiply2 : Product
  Matrix Multiply3 : Product
  Sin1 : Trigonometry
  Sin2 : Trigonometry
  Vector Concatenate1 : Concatenate  NumInputs=3
  F : Outport
  wires:
  Matrix Multiply2/1 -> Gain/1
  Sin1/1 -> Vector Concatenate1/2
  Bx/1 -> Display2/1, Sin1/1, Cos1/1
  Cos1/1 -> Matrix Multiply3/1, Matrix Multiply2/1
  Matrix Multiply3/1 -> Gain1/1
  Cos2/1 -> Matrix Multiply3/2
  By/1 -> Display3/1, Cos2/1, Sin2/1
  Sin2/1 -> Matrix Multiply2/2
  Vector Concatenate1/1 -> Display/1, Matrix Multiply/1  "f_unit"
  Total Force/1 -> Matrix Multiply/2
  Matrix Multiply/1 -> Display1/1, F/1
  Gain/1 -> Vector Concatenate1/1
  Gain1/1 -> Vector Concatenate1/3
